simulink model "SolarRoof"  (R2013b)
settings: Solver=ode3  StartTime=0.0  StopTime=8760  FixedStep=1  RelTol=1e-3
values from neighbouring files (symbols this model uses):
  PVderating = 0.9    [Results.mat]    (also in RunModel.m)
  PVrating = 200    [Results.mat]    (also in RunModel.m)
settings Model: Creator=rogerwong  LastModifiedBy=Nick
settings DataIOCC: SignalLoggingSaveFormat=ModelDataLogs
settings DebuggingCC: UnderspecifiedInitializationDetection=Simplified  MultiTaskDSMMsg=warning  MultiTaskCondExecSysMsg=none  StrictBusMsg=None
settings RTWCC: IncludeERTFirstTime=on
settings GRTTargetCC: CodeReplacementLibrary=None  CPPClassGenCompliant=on

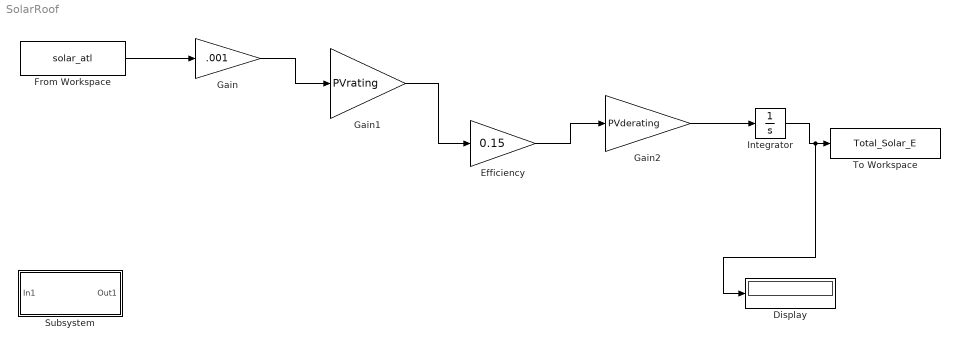
== system SolarRoof ==
  Display : Display
  Efficiency : Gain  Gain=0.15
  From Workspace : FromWorkspace  VariableName=solar_atl  SampleTime=1  Interpolate=off  OutputAfterFinalValue=Holding final value
  Gain : Gain  Gain=.001
  Gain1 : Gain  Gain=PVrating
  Gain2 : Gain  Gain=PVderating
  Integrator : Integrator
  Subsystem : Subsystem
  To Workspace : ToWorkspace  VariableName=Total_Solar_E  SampleTime=-1
  wires:
  Gain/1 -> Gain1/1
  From Workspace/1 -> Gain/1
  Gain1/1 -> Efficiency/1
  Efficiency/1 -> Gain2/1
  Gain2/1 -> Integrator/1
  Integrator/1 -> Display/1, To Workspace/1

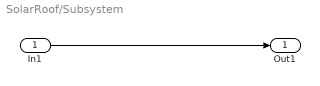
== system SolarRoof/Subsystem ==
  In1 : Inport
  Out1 : Outport
  wires:
  In1/1 -> Out1/1
